simulink model "rc_coder"  (R2019b)
settings: Solver=FixedStepDiscrete  StartTime=0.0  StopTime=Inf  FixedStep=0.025  RelTol=1e-3  EnableMultiTasking=on
PreLoadFcn:
  | mdlname = bdroot;
  | oldFolder = cd(fileparts(which(mdlname)));
  | % cd ..\
  | 
  | load('./bus_type/bus_type.mat');
model workspace (MAT data in the model file):
  ADCDRES : Simulink.Parameter (value not decoded)
  ADCSRES : Simulink.Parameter (value not decoded)
  CLK : Simulink.Parameter (value not decoded)
  EncoderScaler : Simulink.Parameter (value not decoded)
  GearBoxScaler : Simulink.Parameter (value not decoded)
  Kd_T : Simulink.Parameter (value not decoded)
  Kd_theta : Simulink.Parameter (value not decoded)
  Ki_T : Simulink.Parameter (value not decoded)
  Ki_theta : Simulink.Parameter (value not decoded)
  Kp_T : Simulink.Parameter (value not decoded)
  Kp_theta : Simulink.Parameter (value not decoded)
  LowerTempLimitHigh : Simulink.Parameter (value not decoded)
  LowerTempLimitLow : Simulink.Parameter (value not decoded)
  MinMeasurableSpd : Simulink.Parameter (value not decoded)
  ModePWM : Simulink.Parameter (value not decoded)
  ModePosition : Simulink.Parameter (value not decoded)
  ModePrecool : Simulink.Parameter (value not decoded)
  ModeTemp : Simulink.Parameter (value not decoded)
  PWMFreq : Simulink.Parameter (value not decoded)
  QuadratureEncScaler : Simulink.Parameter (value not decoded)
  S1DelaySeconds : Simulink.Parameter (value not decoded)
  S2DelaySeconds : Simulink.Parameter (value not decoded)
  S3DelaySeconds : Simulink.Parameter (value not decoded)
  S4DelaySeconds : Simulink.Parameter (value not decoded)
  SamplingR : Simulink.Parameter (value not decoded)
  StepSize : Simulink.Parameter (value not decoded)
  TErrBand : Simulink.Parameter (value not decoded)
  ThetaErrBand : Simulink.Parameter (value not decoded)
  VADCREF : Simulink.Parameter (value not decoded)
symbols that are objects in the model workspace (value not decoded): ADCDRES, CLK, EncoderScaler, GearBoxScaler, Kd_T, Kd_theta, Ki_T, Ki_theta, Kp_T, Kp_theta, LowerTempLimitHigh, LowerTempLimitLow, MinMeasurableSpd, ModePosition, ModePrecool, ModePWM, ModeTemp, PWMFreq, QuadratureEncScaler, S1DelaySeconds, S2DelaySeconds, S3DelaySeconds, S4DelaySeconds, StepSize, TErrBand, ThetaErrBand
undefined symbols (not defined in the file or in its folder): DiscIntNeverNeededParam, Down, GPTRIP1SEL, GPTRIP2SEL, TZ1, TZ2, Up
libraries: simulink x21, c2802xlib x12, c2837xDlib x10, c280xlib x9, dspstat3 x8, dspfdesign x7, commutil2 x3, c2000lib x2
(part 2 of 4)

== system rc_coder/Controller/Precool Mode ==
  Cmd : Inport
  Action Port : ActionPort  ActionPortLabel=case [ 60 ]:
  Bit to Integer Converter : commutil2/Bit to Integer Converter  nbits=4  bitOrder=MSB first  signedOutputValues=Unsigned  outDtype=Inherit via internal rule  outDtypeSigned=Inherit via internal rule
      settings: SourceProductName=Communications Toolbox
  Bus Selector : BusSelector  OutputSignals=Cmd1,Cmd2,Cmd3,Cmd4
  Constant : Constant  Value=0  OutDataTypeStr=single
  Mux : Mux
  s1 : Outport
  s2 : Outport  Port=2
  s3 : Outport  Port=3
  s4 : Outport  Port=4
  valve : Outport  Port=5
  wires:
  Constant/1 -> s4/1, s3/1, s2/1, s1/1
  Cmd/1 -> Bus Selector/1
  Bit to Integer Converter/1 -> valve/1
  Mux/1 -> Bit to Integer Converter/1
  Bus Selector/1 -> Mux/1  "<Cmd1>"
  Bus Selector/2 -> Mux/2  "<Cmd2>"
  Bus Selector/3 -> Mux/3  "<Cmd3>"
  Bus Selector/4 -> Mux/4  "<Cmd4>"

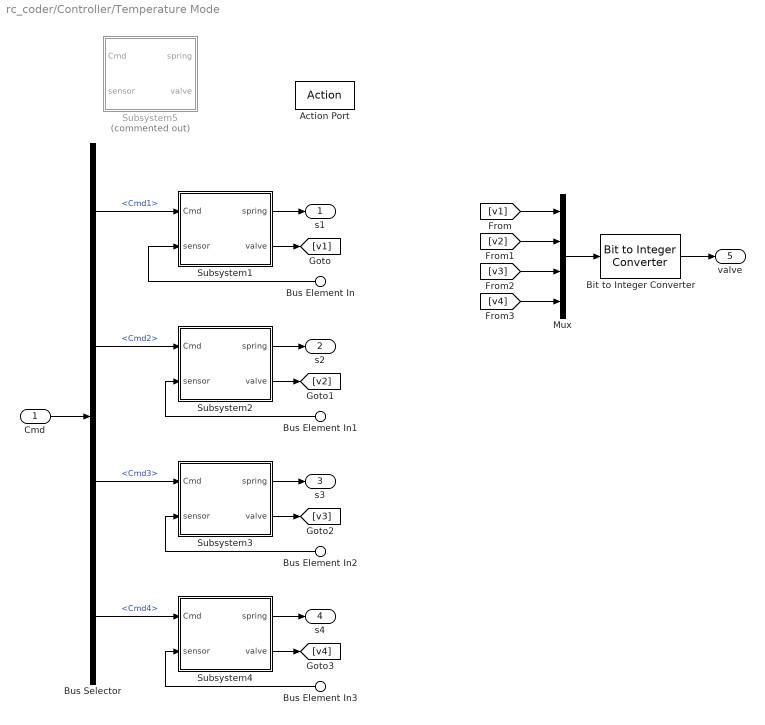
== system rc_coder/Controller/Temperature Mode ==
  Cmd : Inport
  Bus Element In : Inport  Port=2  PortName=feedback  Element=T.T1
  Bus Element In1 : Inport  Port=2  PortName=feedback  Element=T.T2
  Bus Element In2 : Inport  Port=2  PortName=feedback  Element=T.T3
  Bus Element In3 : Inport  Port=2  PortName=feedback  Element=T.T4
  Action Port : ActionPort  ActionPortLabel=case [ 55 ]:
  Bit to Integer Converter : commutil2/Bit to Integer Converter  nbits=4  bitOrder=MSB first  signedOutputValues=Unsigned  outDtype=Inherit via internal rule  outDtypeSigned=Inherit via internal rule
      settings: SourceProductName=Communications Toolbox
  Bus Selector : BusSelector  OutputSignals=Cmd1,Cmd2,Cmd3,Cmd4
  Mux : Mux
  Subsystem1 : Subsystem
  Subsystem2 : Subsystem
  Subsystem3 : Subsystem
  Subsystem4 : Subsystem
  Subsystem5 : Subsystem  Commented=on
  s1 : Outport
  s2 : Outport  Port=2
  s3 : Outport  Port=3
  s4 : Outport  Port=4
  valve : Outport  Port=5
  wires:
  Cmd/1 -> Bus Selector/1
  Subsystem2/1(spring) -> s2/1
  Subsystem3/1(spring) -> s3/1
  Bus Element In3/1 -> Subsystem4/2(sensor)
  Bus Selector/4 -> Subsystem4/1(Cmd)  "<Cmd4>"
  Subsystem4/1(spring) -> s4/1
  Bus Element In2/1 -> Subsystem3/2(sensor)
  Bus Selector/3 -> Subsystem3/1(Cmd)  "<Cmd3>"
  Mux/1 -> Bit to Integer Converter/1
  [v1] -> Mux/1
  [v2] -> Mux/2
  [v3] -> Mux/3
  [v4] -> Mux/4
  Bit to Integer Converter/1 -> valve/1
  Bus Selector/1 -> Subsystem1/1(Cmd)  "<Cmd1>"
  Bus Element In/1 -> Subsystem1/2(sensor)
  Subsystem1/1(spring) -> s1/1
  Subsystem1/2(valve) -> [v1]
  Bus Selector/2 -> Subsystem2/1(Cmd)  "<Cmd2>"
  Subsystem2/2(valve) -> [v2]
  Bus Element In1/1 -> Subsystem2/2(sensor)
  Subsystem3/2(valve) -> [v3]
  Subsystem4/2(valve) -> [v4]

== system rc_coder/Data Uploading/Subsystem1 ==
  In1 : Inport
  Constant2 : Constant  Value=f
  Data Type Conversion : DataTypeConversion  OutDataTypeStr=int32
  Product1 : Product
  Rounding Function : Rounding  Operator=round
  Out1 : Outport
  wires:
  Rounding Function/1 -> Data Type Conversion/1
  Constant2/1 -> Product1/2
  In1/1 -> Product1/1
  Product1/1 -> Rounding Function/1
  Data Type Conversion/1 -> Out1/1

== system rc_coder/Data Uploading/Subsystem2 ==
  In1 : Inport
  Constant2 : Constant  Value=f
  Data Type Conversion : DataTypeConversion  OutDataTypeStr=int32
  Product1 : Product
  Rounding Function : Rounding  Operator=round
  Out1 : Outport
  wires:
  Data Type Conversion/1 -> Out1/1
  Product1/1 -> Rounding Function/1
  In1/1 -> Product1/1
  Constant2/1 -> Product1/2
  Rounding Function/1 -> Data Type Conversion/1

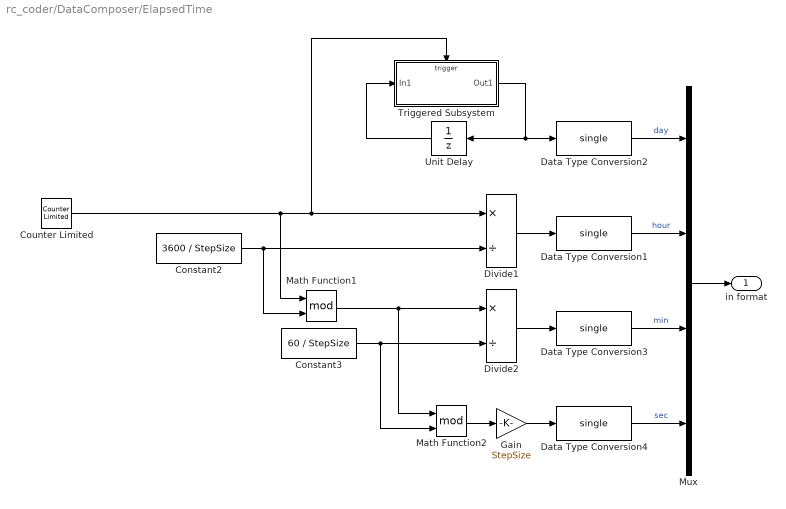
== system rc_coder/DataComposer/ElapsedTime ==
  Constant2 : Constant  Value=3600 / StepSize  OutDataTypeStr=uint32
  Constant3 : Constant  Value=60 / StepSize  OutDataTypeStr=uint32
  Counter Limited : simulink/Sources/Counter Limited  uplimit=1 / StepSize * 60 * 60 * 24  tsamp=-1
  Data Type Conversion{1..4} (4 alike) : DataTypeConversion  OutDataTypeStr=single
  Divide1 : Product  Inputs=*/  OutDataTypeStr=uint8
  Divide2 : Product  Inputs=*/  OutDataTypeStr=uint8
  Gain : Gain  Gain=StepSize  OutDataTypeStr=single
  Math Function1 : Math  Operator=mod  SignedPower=off  SaturateOnIntegerOverflow=on
  Math Function2 : Math  Operator=mod  SignedPower=off  SaturateOnIntegerOverflow=on
  Mux : Mux
  Triggered Subsystem : Subsystem  TreatAsAtomicUnit=on
  Unit Delay : UnitDelay  SampleTime=-1  HasFrameUpgradeWarning=on
  in format : Outport
  wires:
  Counter Limited/1 -> Divide1/1, Triggered Subsystem/Trigger, Math Function1/1
  Divide1/1 -> Data Type Conversion1/1
  Divide2/1 -> Data Type Conversion3/1
  Constant2/1 -> Math Function1/2, Divide1/2
  Math Function1/1 -> Divide2/1, Math Function2/1
  Data Type Conversion2/1 -> Mux/1  "day"
  Data Type Conversion1/1 -> Mux/2  "hour"
  Data Type Conversion3/1 -> Mux/3  "min"
  Data Type Conversion4/1 -> Mux/4  "sec"
  Math Function2/1 -> Gain/1
  Constant3/1 -> Divide2/2, Math Function2/2
  Mux/1 -> in format/1
  Triggered Subsystem/1(Out1) -> Data Type Conversion2/1, Unit Delay/1
  Unit Delay/1 -> Triggered Subsystem/1(In1)
  Gain/1 -> Data Type Conversion4/1

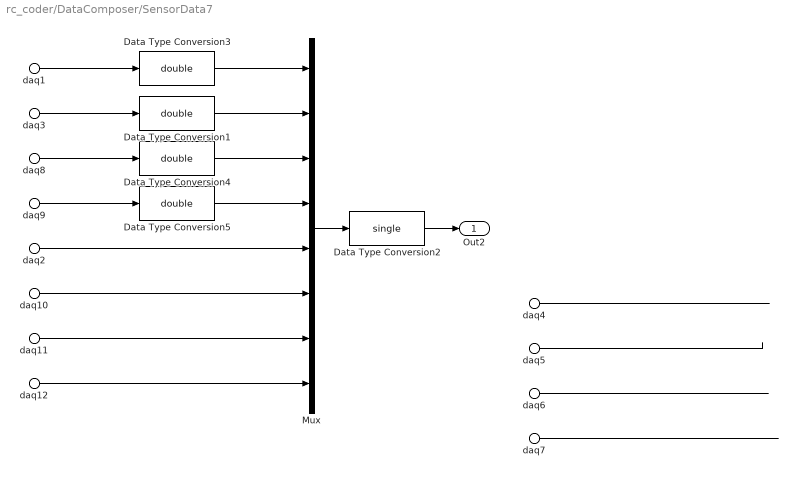
== system rc_coder/DataComposer/SensorData7 ==
  daq1 : Inport  PortName=daq  Element=ENC.PosA
  daq3 : Inport  PortName=daq  Element=ENC.SpdA
  daq8 : Inport  PortName=daq  Element=ENC.PosB
  daq9 : Inport  PortName=daq  Element=ENC.SpdB
  daq2 : Inport  PortName=daq  Element=T.T1
  daq10 : Inport  PortName=daq  Element=T.T2
  daq11 : Inport  PortName=daq  Element=T.T3
  daq12 : Inport  PortName=daq  Element=T.T4
  daq4 : Inport  PortName=daq  Element=I.current1
  daq5 : Inport  PortName=daq  Element=I.current2
  daq6 : Inport  PortName=daq  Element=I.current3
  daq7 : Inport  PortName=daq  Element=I.current4
  Data Type Conversion{1,3..5} (4 alike) : DataTypeConversion  OutDataTypeStr=double
  Data Type Conversion2 : DataTypeConversion  OutDataTypeStr=single
  Mux : Mux  Inputs=8
  Out2 : Outport
  wires:
  daq3/1 -> Data Type Conversion1/1
  Data Type Conversion1/1 -> Mux/2
  Data Type Conversion3/1 -> Mux/1
  daq2/1 -> Mux/5
  daq1/1 -> Data Type Conversion3/1
  Mux/1 -> Data Type Conversion2/1
  daq4/1 -> ?
  daq5/1 -> ?
  daq6/1 -> ?
  daq7/1 -> ?
  Data Type Conversion2/1 -> Out2/1
  daq8/1 -> Data Type Conversion4/1
  Data Type Conversion4/1 -> Mux/3
  daq9/1 -> Data Type Conversion5/1
  Data Type Conversion5/1 -> Mux/4
  daq10/1 -> Mux/6
  daq11/1 -> Mux/7
  daq12/1 -> Mux/8

== system rc_coder/Receive/Triggered Subsystem2 ==
  SCIA RCV Interrupt : TriggerPort  TriggerType=function-call  VariantControl=Variant
  SCI Receive : c280xlib/SCI Receive  sciModule=B  dataHead=''  dataTail=''  dataType=single  dataDim=5  initValue=0  errOption=Output the last received value  errValue=0  sampleTime=-1  outputStatus=off  postInterrupt=on  numFifo=1
      settings: SourceProductName=Embedded Coder Support Package for Texas Instruments C2000 Processors  SourceProductBaseCode=TIC2000
  Serial Command : Outport
  wires:
  SCI Receive/1 -> Serial Command/1

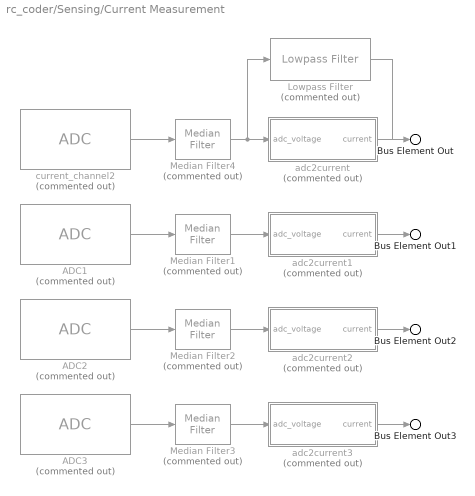
== system rc_coder/Sensing/Current Measurement ==
  ADC1 : c2802xlib/ADC  Commented=on  blkParamProc=C2000_Type4  ADCModule=B  samplingMode=Single sample mode  ADCResolution=16-bit (Differential inputs)  useSOC1=SOC5  useSOC2=SOC0_SOC1  SOCAcquisitionWindow=15  SOCTriggerSource=Software  SOCInterruptTrigger=No ADCINT  Ts=-1  dType=double  postInterrupt=off  interruptSel=ADCINT1  ADCINTContinuous=on  endma=off  chdma=1  conv1=ADCINA0  conv2=ADCINA0 and ADCINB0  conv1_Type4=ADCIN5  conv2_Type4=ADCIN4 and ADCIN5
      settings: SourceProductName=Embedded Coder Support Package for Texas Instruments C2000 Processors
  ADC2 : c2802xlib/ADC  Commented=on  blkParamProc=C2000_Type4  ADCModule=C  samplingMode=Single sample mode  ADCResolution=16-bit (Differential inputs)  useSOC1=SOC5  useSOC2=SOC0_SOC1  SOCAcquisitionWindow=15  SOCTriggerSource=Software  SOCInterruptTrigger=No ADCINT  Ts=-1  dType=double  postInterrupt=off  interruptSel=ADCINT1  ADCINTContinuous=on  endma=off  chdma=1  conv1=ADCINA0  conv2=ADCINA0 and ADCINB0  conv1_Type4=ADCIN5  conv2_Type4=ADCIN4 and ADCIN5
      settings: SourceProductName=Embedded Coder Support Package for Texas Instruments C2000 Processors
  ADC3 : c2802xlib/ADC  Commented=on  blkParamProc=C2000_Type4  ADCModule=A  samplingMode=Single sample mode  ADCResolution=16-bit (Differential inputs)  useSOC1=SOC4  useSOC2=SOC0_SOC1  SOCAcquisitionWindow=15  SOCTriggerSource=Software  SOCInterruptTrigger=No ADCINT  Ts=-1  dType=double  postInterrupt=off  interruptSel=ADCINT1  ADCINTContinuous=on  endma=off  chdma=1  conv1=ADCINA0  conv2=ADCINA0 and ADCINB0  conv1_Type4=ADCIN4  conv2_Type4=ADCIN0 and ADCIN1
      settings: SourceProductName=Embedded Coder Support Package for Texas Instruments C2000 Processors
  Lowpass Filter : dspfdesign/Lowpass Filter  Commented=on  FilterType=FIR  DesignForMinimumOrder=on  FilterOrder=50  PassbandFrequency=2  StopbandFrequency=5  PassbandRipple=0.1  StopbandAttenuation=80  InheritSampleRate=off  SampleRate=1000  SimulateUsing=Code generation  roundingMode=Floor  coeffsDataTypeStr=fixdt(1,16)
  Median Filter1 : dspstat3/Median Filter  Commented=on  WindowLength=5  SimulateUsing=Code generation
      settings: SourceProductName=DSP System Toolbox  SourceProductBaseCode=DS
  Median Filter2 : dspstat3/Median Filter  Commented=on  WindowLength=5  SimulateUsing=Code generation
      settings: SourceProductName=DSP System Toolbox  SourceProductBaseCode=DS
  Median Filter3 : dspstat3/Median Filter  Commented=on  WindowLength=5  SimulateUsing=Code generation
      settings: SourceProductName=DSP System Toolbox  SourceProductBaseCode=DS
  Median Filter4 : dspstat3/Median Filter  Commented=on  WindowLength=10  SimulateUsing=Code generation
      settings: SourceProductName=DSP System Toolbox  SourceProductBaseCode=DS
  adc2current : Subsystem  Commented=on
  adc2current1 : Subsystem  Commented=on
  adc2current2 : Subsystem  Commented=on
  adc2current3 : Subsystem  Commented=on
  current_channel2 : c2802xlib/ADC  Commented=on  blkParamProc=C2000_Type4  ADCModule=A  samplingMode=Single sample mode  ADCResolution=16-bit (Differential inputs)  useSOC1=SOC2  useSOC2=SOC0_SOC1  SOCAcquisitionWindow=15  SOCTriggerSource=Software  SOCInterruptTrigger=No ADCINT  Ts=-1  dType=double  postInterrupt=off  interruptSel=ADCINT1  ADCINTContinuous=on  endma=off  chdma=1  conv1=ADCINA0  conv2=ADCINA0 and ADCINB0  conv1_Type4=ADCIN5  conv2_Type4=ADCIN4 and ADCIN5
      settings: SourceProductName=Embedded Coder Support Package for Texas Instruments C2000 Processors
  Bus Element Out : Outport  PortName=OutBus  Element=current1
  Bus Element Out1 : Outport  PortName=OutBus  Element=current2
  Bus Element Out2 : Outport  PortName=OutBus  Element=current3
  Bus Element Out3 : Outport  PortName=OutBus  Element=current4
  wires:
  ADC1/1 -> Median Filter1/1
  current_channel2/1 -> Median Filter4/1
  ADC2/1 -> Median Filter2/1
  ADC3/1 -> Median Filter3/1
  adc2current1/1(current) -> Bus Element Out1/1
  adc2current2/1(current) -> Bus Element Out2/1
  adc2current3/1(current) -> Bus Element Out3/1
  Median Filter1/1 -> adc2current1/1(adc_voltage)
  Median Filter2/1 -> adc2current2/1(adc_voltage)
  Median Filter3/1 -> adc2current3/1(adc_voltage)
  Median Filter4/1 -> Lowpass Filter/1, adc2current/1(adc_voltage)
  adc2current/1(current) -> ?
  Lowpass Filter/1 -> Bus Element Out/1

== system rc_coder/Sensing/Incremental Encoder ==
  CalcSpd : Subsystem
  CalcSpd1 : Subsystem
  Gain1 : Gain  Gain=360 / (EncoderScaler * GearBoxScaler * QuadratureEncScaler)
  Gain2 : Gain  Gain=360 / (EncoderScaler * GearBoxScaler * QuadratureEncScaler)
  eCAP : c280xlib/eCAP  operatingMode=eCAP  selectCAPx=eCAP1  offsetValue=0  counterSynIn=off  enableCounter=off  syncOutput=Disabled  sampleTime=-1  eventPrescaler=0  selectMode=Continuous  enableOneShot=off  stopValue=Capture Event 1  resetEv1Ts=on  ev1Polarity=Rising Edge  resetEv2Ts=off  ev2Polarity=Rising Edge  resetEv3Ts=off  ev3Polarity=Rising Edge  resetEv4Ts=off  ev4Polarity=Rising Edge  tSCntrDataType=uint32  capEvFlag=off  capFlagDataType=uint16  overFlowFlag=on  overFlowFlagDataType=uint32  periodUnit=Seconds  periodSource=Specify via dialog  waveformPeriod=0.001  dutyUnit=Percentages  dutySource=Specify via dialog  dutyCycle=50  outputPolarity=Active High  enableCEVT1Int=off  enableCEVT2Int=off  enableCEVT3Int=off  enableCEVT4Int=off  enableCTROVFInt=off  enablePRDInt=off  enableCMPInt=off
      settings: SourceProductName=Embedded Coder Support Package for Texas Instruments C2000 Processors  SourceProductBaseCode=TIC2000
  eCAP1 : c280xlib/eCAP  operatingMode=eCAP  selectCAPx=eCAP4  offsetValue=0  counterSynIn=off  enableCounter=off  syncOutput=Disabled  sampleTime=-1  eventPrescaler=0  selectMode=Continuous  enableOneShot=off  stopValue=Capture Event 1  resetEv1Ts=on  ev1Polarity=Rising Edge  resetEv2Ts=off  ev2Polarity=Rising Edge  resetEv3Ts=off  ev3Polarity=Rising Edge  resetEv4Ts=off  ev4Polarity=Rising Edge  tSCntrDataType=uint32  capEvFlag=off  capFlagDataType=uint16  overFlowFlag=on  overFlowFlagDataType=uint32  periodUnit=Seconds  periodSource=Specify via dialog  waveformPeriod=0.001  dutyUnit=Percentages  dutySource=Specify via dialog  dutyCycle=50  outputPolarity=Active High  enableCEVT1Int=off  enableCEVT2Int=off  enableCEVT3Int=off  enableCEVT4Int=off  enableCTROVFInt=off  enablePRDInt=off  enableCMPInt=off
      settings: SourceProductName=Embedded Coder Support Package for Texas Instruments C2000 Processors  SourceProductBaseCode=TIC2000
  eQEP : c280xlib/eQEP  useModule=eQEP1  pcInputmode=Quadrature-count  externalClockrate=2x resolution: Count the rising/falling edge  swapPolarityselection=Clockwise  qdfOutputport=on  qapPolarityselection=off  qbpPolarityselection=off  qipPolarityselection=off  qspPolarityselection=off  igatePolarityselection=off  sampleTime=-1  pcOutputport=on  pcMaximumvalue=4294967295  indexInitializationcheck=off  indexInitializationevent=Rising edge  strobeInitializationcheck=off  strobeInitializationevent=Rising edge  softwareInitializationcheck=off  softwareInitializationsource=Set to init value at start up  softwareInitializationmode=on  pcInitialvalue=2147483648  pcResetmode=Reset on an index event  ieloutputport=off  indexEventlatch=Rising edge  seloutputport=off  strobeEventlatch=Rising edge  pcefOutputport=off  enableEqepcapture=off  qctmrOutputport=off  qcprdOutputport=off  captureTimerprescaler=128  upEventprescaler=2  overflowErrorflag=off  directionErrorflag=off  captureTimerposition=On position counter read  unitTimerperiod=100000000  captureTimerlatch=off  capturePeriodlatch=on  positionCounterlatch=off  soenPolarityselection=off  spselPolarityselection=Index pin is used for sync output  compareValuesource=Specify via dialog  shadowMode=Load on QPOSCNT=0  compareValue=4294967295  syncOutputwidth=1  polaritySyncoutput=Active high  watchdogEnable=off  watchdogTimer=65535  outport1Datatype=auto  outport2Datatype=int32  outport3Datatype=auto  outport4Datatype=auto  outport5Datatype=auto  outport6Datatype=auto  outport7Datatype=auto  outport8Datatype=auto  outport9Datatype=auto  outport10Datatype=auto  outport11Datatype=auto  outport12Datatype=auto  eqepinterrupt_pce=off  eqepinterrupt_qpe=off  eqepinterrupt_qdc=off  eqepinterrupt_wto=off  eqepinterrupt_pcu=off  eqepinterrupt_pco=off  eqepinterrupt_pcr=off  eqepinterrupt_pcm=off  eqepinterrupt_sel=off  eqepinterrupt_iel=off  eqepinterrupt_uto=off  pheOutputport=off  watchdogOutputport=off  outport13Datatype=auto  outport14Datatype=auto
      settings: SourceProductName=Embedded Coder Support Package for Texas Instruments C2000 Processors  SourceProductBaseCode=TIC2000
  eQEP1 : c280xlib/eQEP  useModule=eQEP2  pcInputmode=Quadrature-count  externalClockrate=2x resolution: Count the rising/falling edge  swapPolarityselection=Clockwise  qdfOutputport=on  qapPolarityselection=off  qbpPolarityselection=off  qipPolarityselection=off  qspPolarityselection=off  igatePolarityselection=off  sampleTime=-1  pcOutputport=on  pcMaximumvalue=4294967295  indexInitializationcheck=off  indexInitializationevent=Rising edge  strobeInitializationcheck=off  strobeInitializationevent=Rising edge  softwareInitializationcheck=off  softwareInitializationsource=Set to init value at start up  softwareInitializationmode=on  pcInitialvalue=2147483648  pcResetmode=Reset on an index event  ieloutputport=off  indexEventlatch=Rising edge  seloutputport=off  strobeEventlatch=Rising edge  pcefOutputport=off  enableEqepcapture=off  qctmrOutputport=off  qcprdOutputport=on  captureTimerprescaler=128  upEventprescaler=128  overflowErrorflag=off  directionErrorflag=off  captureTimerposition=On position counter read  unitTimerperiod=100000000  captureTimerlatch=off  capturePeriodlatch=off  positionCounterlatch=off  soenPolarityselection=off  spselPolarityselection=Index pin is used for sync output  compareValuesource=Specify via dialog  shadowMode=Load on QPOSCNT=0  compareValue=4294967295  syncOutputwidth=1  polaritySyncoutput=Active high  watchdogEnable=off  watchdogTimer=65535  outport1Datatype=auto  outport2Datatype=int32  outport3Datatype=auto  outport4Datatype=auto  outport5Datatype=auto  outport6Datatype=auto  outport7Datatype=auto  outport8Datatype=auto  outport9Datatype=auto  outport10Datatype=auto  outport11Datatype=auto  outport12Datatype=auto  eqepinterrupt_pce=off  eqepinterrupt_qpe=off  eqepinterrupt_qdc=off  eqepinterrupt_wto=off  eqepinterrupt_pcu=off  eqepinterrupt_pco=off  eqepinterrupt_pcr=off  eqepinterrupt_pcm=off  eqepinterrupt_sel=off  eqepinterrupt_iel=off  eqepinterrupt_uto=off  pheOutputport=off  watchdogOutputport=off  outport13Datatype=auto  outport14Datatype=auto
      settings: SourceProductName=Embedded Coder Support Package for Texas Instruments C2000 Processors  SourceProductBaseCode=TIC2000
  Bus Element Out : Outport  PortName=OutBus  Element=PosA
  Bus Element Out1 : Outport  PortName=OutBus  Element=SpdA
  Bus Element Out2 : Outport  PortName=OutBus  Element=PosB
  Bus Element Out3 : Outport  PortName=OutBus  Element=SpdB
  wires:
  eQEP/2 -> Gain1/1, CalcSpd/2(qposcnt)
  Gain1/1 -> Bus Element Out/1
  eQEP1/1 -> CalcSpd1/1(dir)
  eQEP1/2 -> Gain2/1, CalcSpd1/2(qposcnt)
  Gain2/1 -> Bus Element Out2/1
  CalcSpd/1(speed) -> Bus Element Out1/1
  eCAP/1 -> CalcSpd/3(qcprd)
  eCAP/2 -> CalcSpd/4(overflow)
  eQEP/1 -> CalcSpd/1(dir)
  CalcSpd1/1(speed) -> Bus Element Out3/1
  eCAP1/1 -> CalcSpd1/3(qcprd)
  eCAP1/2 -> CalcSpd1/4(overflow)

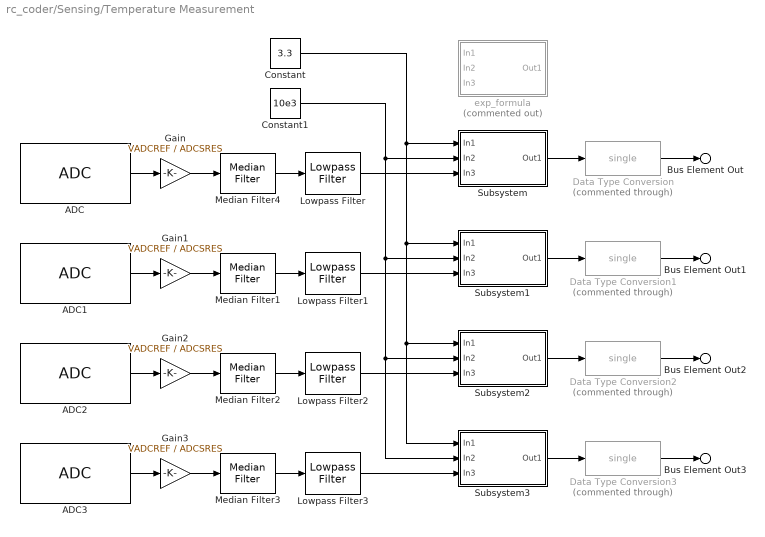
== system rc_coder/Sensing/Temperature Measurement ==
  ADC : c2802xlib/ADC  blkParamProc=C2000_Type4  ADCModule=C  samplingMode=Single sample mode  ADCResolution=12-bit (Single-ended input)  useSOC1=SOC3  useSOC2=SOC0_SOC1  SOCAcquisitionWindow=15  SOCTriggerSource=Software  SOCInterruptTrigger=No ADCINT  Ts=-1  dType=double  postInterrupt=off  interruptSel=ADCINT1  ADCINTContinuous=on  endma=off  chdma=1  conv1=ADCINA0  conv2=ADCINA0 and ADCINB0  conv1_Type4=ADCIN3  conv2_Type4=ADCIN2 and ADCIN3
      settings: SourceProductName=Embedded Coder Support Package for Texas Instruments C2000 Processors
  ADC1 : c2802xlib/ADC  blkParamProc=C2000_Type4  ADCModule=B  samplingMode=Single sample mode  ADCResolution=12-bit (Single-ended input)  useSOC1=SOC3  useSOC2=SOC0_SOC1  SOCAcquisitionWindow=15  SOCTriggerSource=Software  SOCInterruptTrigger=No ADCINT  Ts=-1  dType=double  postInterrupt=off  interruptSel=ADCINT1  ADCINTContinuous=on  endma=off  chdma=1  conv1=ADCINA0  conv2=ADCINA0 and ADCINB0  conv1_Type4=ADCIN3  conv2_Type4=ADCIN0 and ADCIN1
      settings: SourceProductName=Embedded Coder Support Package for Texas Instruments C2000 Processors
  ADC2 : c2802xlib/ADC  blkParamProc=C2000_Type4  ADCModule=A  samplingMode=Single sample mode  ADCResolution=12-bit (Single-ended input)  useSOC1=SOC3  useSOC2=SOC0_SOC1  SOCAcquisitionWindow=15  SOCTriggerSource=Software  SOCInterruptTrigger=No ADCINT  Ts=-1  dType=double  postInterrupt=off  interruptSel=ADCINT1  ADCINTContinuous=on  endma=off  chdma=1  conv1=ADCINA0  conv2=ADCINA0 and ADCINB0  conv1_Type4=ADCIN3  conv2_Type4=ADCIN0 and ADCIN1
      settings: SourceProductName=Embedded Coder Support Package for Texas Instruments C2000 Processors
  ADC3 : c2802xlib/ADC  blkParamProc=C2000_Type4  ADCModule=C  samplingMode=Single sample mode  ADCResolution=12-bit (Single-ended input)  useSOC1=SOC2  useSOC2=SOC0_SOC1  SOCAcquisitionWindow=15  SOCTriggerSource=Software  SOCInterruptTrigger=No ADCINT  Ts=-1  dType=double  postInterrupt=off  interruptSel=ADCINT1  ADCINTContinuous=on  endma=off  chdma=1  conv1=ADCINA0  conv2=ADCINA0 and ADCINB0  conv1_Type4=ADCIN2  conv2_Type4=ADCIN0 and ADCIN1
      settings: SourceProductName=Embedded Coder Support Package for Texas Instruments C2000 Processors
  Constant : Constant  Value=3.3  OutDataTypeStr=double
  Constant1 : Constant  Value=10e3  OutDataTypeStr=double
  Data Type Conversion{,1..3} (4 alike) : DataTypeConversion  Commented=through  OutDataTypeStr=single
  Gain{,1..3} (4 alike) : Gain  Gain=VADCREF / ADCSRES
  Lowpass Filter{,1..3} (4 alike) : dspfdesign/Lowpass Filter  FilterType=IIR  DesignForMinimumOrder=on  FilterOrder=50  PassbandFrequency=10  StopbandFrequency=19  PassbandRipple=0.1  StopbandAttenuation=80  InheritSampleRate=off  SampleRate=1/StepSize  SimulateUsing=Code generation  roundingMode=Floor  coeffsDataTypeStr=fixdt(1,16)
  Median Filter{1..4} (4 alike) : dspstat3/Median Filter  WindowLength=5  SimulateUsing=Code generation
      settings: SourceProductName=DSP System Toolbox  SourceProductBaseCode=DS
  Subsystem : Subsystem
      mask Display:
      | disp('u2T');
      | port_label('input', 1, 'excitation');
      | port_label('input', 2, 'R');
      | port_label('input', 3, 'u');
  Subsystem1 : Subsystem
      mask Display:
      | disp('u2T');
      | port_label('input', 1, 'excitation');
      | port_label('input', 2, 'R');
      | port_label('input', 3, 'u');
  Subsystem2 : Subsystem
      mask Display:
      | disp('u2T');
      | port_label('input', 1, 'excitation');
      | port_label('input', 2, 'R');
      | port_label('input', 3, 'u');
  Subsystem3 : Subsystem
      mask Display:
      | disp('u2T');
      | port_label('input', 1, 'excitation');
      | port_label('input', 2, 'R');
      | port_label('input', 3, 'u');
  exp_formula : Subsystem  Commented=on
      mask Display:
      | disp('u2T');
      | port_label('input', 1, 'excitation');
      | port_label('input', 2, 'R');
      | port_label('input', 3, 'u');
  Bus Element Out : Outport  PortName=OutBus  Element=T1
  Bus Element Out1 : Outport  PortName=OutBus  Element=T2
  Bus Element Out2 : Outport  PortName=OutBus  Element=T3
  Bus Element Out3 : Outport  PortName=OutBus  Element=T4
  wires:
  Subsystem1/1(Out1) -> Data Type Conversion1/1
  Gain1/1 -> Median Filter1/1
  Subsystem2/1(Out1) -> Data Type Conversion2/1
  Gain2/1 -> Median Filter2/1
  Median Filter1/1 -> Lowpass Filter1/1
  Median Filter2/1 -> Lowpass Filter2/1
  ADC/1 -> Gain/1
  Median Filter4/1 -> Lowpass Filter/1
  Median Filter3/1 -> Lowpass Filter3/1
  Constant1/1 -> Subsystem1/2(In2), Subsystem3/2(In2), Subsystem2/2(In2), Subsystem/2(In2)
  Gain3/1 -> Median Filter3/1
  Subsystem3/1(Out1) -> Data Type Conversion3/1
  Lowpass Filter/1 -> Subsystem/3(In3)
  Lowpass Filter1/1 -> Subsystem1/3(In3)
  Lowpass Filter2/1 -> Subsystem2/3(In3)
  Lowpass Filter3/1 -> Subsystem3/3(In3)
  Gain/1 -> Median Filter4/1
  ADC3/1 -> Gain3/1
  ADC2/1 -> Gain2/1
  ADC1/1 -> Gain1/1
  Data Type Conversion/1 -> Bus Element Out/1
  Data Type Conversion1/1 -> Bus Element Out1/1
  Data Type Conversion2/1 -> Bus Element Out2/1
  Data Type Conversion3/1 -> Bus Element Out3/1
  Subsystem/1(Out1) -> Data Type Conversion/1
  Constant/1 -> Subsystem/1(In1), Subsystem1/1(In1), Subsystem3/1(In1), Subsystem2/1(In1)

== system rc_coder/SerialCommInterface1/Triggered Subsystem1 ==
  TX : Inport
  SCIA RCV Interrupt : TriggerPort  TriggerType=function-call  VariantControl=Variant
  Mux : Mux  Inputs=2
  SCI Receive : c280xlib/SCI Receive  sciModule=A  dataHead=''  dataTail=''  dataType=single  dataDim=1  initValue=0  errOption=Output the last received value  errValue=0  sampleTime=-1  outputStatus=off  postInterrupt=on  numFifo=1
      settings: SourceProductName=Embedded Coder Support Package for Texas Instruments C2000 Processors  SourceProductBaseCode=TIC2000
  SCI Transmit : c280xlib/SCI Transmit  sciModule=A  dataHead=''  dataTail=''  postInterrupt=off  numFifo=1
      settings: SourceProductName=Embedded Coder Support Package for Texas Instruments C2000 Processors
  Serial Command : Outport
  wires:
  TX/1 -> Mux/2
  Mux/1 -> SCI Transmit/1
  SCI Receive/1 -> Mux/1, Serial Command/1

== system rc_coder/Transmit/DataFlowSwitch ==
  status : Inport
  If Action Subsystem1 : Subsystem  TreatAsAtomicUnit=on
  If Action Subsystem2 : Subsystem  TreatAsAtomicUnit=on
  If1 : If  IfExpression=(u1 == ModePosition) | (u1 == ModePrecool) | (u1 == ModePWM) | (u1 == ModeTemp)
  If2 : If  Commented=on  IfExpression=(u1 == ModePosition) | (u1 == ModePrecool)
  Merge : Merge
  switch : Outport
  wires:
  If Action Subsystem1/1(Out1) -> Merge/1
  If Action Subsystem2/1(Out1) -> Merge/2
  If1/2 -> If Action Subsystem2/Action
  Merge/1 -> switch/1
  If1/1 -> If Action Subsystem1/Action
  status/1 -> If1/1, If Action Subsystem2/1(In1)

== system rc_coder/Transmit/If Action Subsystem ==
  received : Inport
  status : Inport  Port=2
  data : Inport  Port=3
  Action Port : ActionPort  ActionPortLabel=if(u1 == 1)
  Mux : Mux  Inputs=3
  SCI Transmit : c280xlib/SCI Transmit  sciModule=B  dataHead=''  dataTail=''  postInterrupt=off  numFifo=1
      settings: SourceProductName=Embedded Coder Support Package for Texas Instruments C2000 Processors
  wires:
  status/1 -> Mux/2
  data/1 -> Mux/3
  Mux/1 -> SCI Transmit/1
  received/1 -> Mux/1

== system rc_coder/Controller/Position Mode/PID ==
  note: integrator and derivative should be of discrete type due to descrete solver
  In1 : Inport
  In2 : Inport  Port=2
  In3 : Inport  Port=3
  In4 : Inport  Port=4
  Abs : Abs
  Add : Sum  Inputs=+++
  Constant1 : Constant
  Constant5 : Constant  Value=0
  Discrete Derivative : simulink/Discrete/Discrete Derivative  gainval=1.0  ICPrevScaledInput=0.0  OutMin=[]  OutMax=[]  OutDataType=fixdt(1, 16)  OutScaling=2^-10  DoSatur=off
  Discrete-Time Integrator : DiscreteIntegrator  SampleTime=-1  LimitOutput=on  UpperSaturationLimit=0.5  LowerSaturationLimit=-0.5  ICPrevOutput=DiscIntNeverNeededParam  ICPrevScaledInput=DiscIntNeverNeededParam
  Product{,1..3} (4 alike) : Product
  Switch2 : Switch  Criteria=u2 > Threshold  Threshold=ThetaErrBand
  Out1 : Outport
  wires:
  Add/1 -> Product3/2
  Discrete Derivative/1 -> Add/3
  Discrete-Time Integrator/1 -> Add/2
  Product/1 -> Discrete-Time Integrator/1
  Product1/1 -> Discrete Derivative/1
  Product2/1 -> Add/1
  In1/1 -> Abs/1, Product2/1, Product/1, Product1/1
  Abs/1 -> Switch2/2
  Constant5/1 -> Switch2/3
  Product3/1 -> Out1/1
  Constant1/1 -> Switch2/1
  Switch2/1 -> Product3/1
  In2/1 -> Product2/2
  In3/1 -> Product/2
  In4/1 -> Product1/2

== system rc_coder/Controller/Position Mode/PID1 ==
  note: integrator and derivative should be of discrete type due to descrete solver
  In1 : Inport
  In2 : Inport  Port=2
  In3 : Inport  Port=3
  In4 : Inport  Port=4
  Abs : Abs
  Add : Sum  Inputs=+++
  Constant1 : Constant
  Constant5 : Constant  Value=0
  Discrete Derivative : simulink/Discrete/Discrete Derivative  gainval=1.0  ICPrevScaledInput=0.0  OutMin=[]  OutMax=[]  OutDataType=fixdt(1, 16)  OutScaling=2^-10  DoSatur=off
  Discrete-Time Integrator : DiscreteIntegrator  SampleTime=-1  LimitOutput=on  UpperSaturationLimit=0.5  LowerSaturationLimit=-0.5  ICPrevOutput=DiscIntNeverNeededParam  ICPrevScaledInput=DiscIntNeverNeededParam
  Product{,1..3} (4 alike) : Product
  Switch2 : Switch  Criteria=u2 > Threshold  Threshold=ThetaErrBand
  Out1 : Outport
  wires:
  In4/1 -> Product1/2
  In3/1 -> Product/2
  In2/1 -> Product2/2
  Switch2/1 -> Product3/1
  Constant1/1 -> Switch2/1
  Product3/1 -> Out1/1
  Constant5/1 -> Switch2/3
  Abs/1 -> Switch2/2
  In1/1 -> Product1/1, Product/1, Product2/1, Abs/1
  Product2/1 -> Add/1
  Product1/1 -> Discrete Derivative/1
  Product/1 -> Discrete-Time Integrator/1
  Discrete-Time Integrator/1 -> Add/2
  Discrete Derivative/1 -> Add/3
  Add/1 -> Product3/2

== system rc_coder/Controller/Position Mode/Subsystem1 ==
  Cmd : Inport
  sensor : Inport  Port=2
  Constant : Constant  Value=Kp_T
  Constant1 : Constant  Value=Ki_T
  Constant2 : Constant  Value=Kd_T
  Data Type Conversion : DataTypeConversion
  PID : Subsystem
  Saturation : Saturate  UpperLimit=60  LowerLimit=-20
  Subsystem : Subsystem
  Sum : Sum  Inputs=|+-
  spring : Outport
  valve : Outport  Port=2
  wires:
  Constant1/1 -> PID/3(Ki)
  Constant2/1 -> PID/4(Kd)
  Constant/1 -> PID/2(Kp)
  Cmd/1 -> Saturation/1
  Subsystem/1(heating) -> spring/1
  Subsystem/2(cooling) -> valve/1
  Data Type Conversion/1 -> PID/1(e)
  Saturation/1 -> Sum/1
  sensor/1 -> Sum/2
  PID/1(u) -> Subsystem/1(u)
  Sum/1 -> Data Type Conversion/1

== system rc_coder/Controller/Position Mode/Subsystem2 ==
  Cmd : Inport
  sensor : Inport  Port=2
  Constant : Constant  Value=Kp_T
  Constant1 : Constant  Value=Ki_T
  Constant2 : Constant  Value=Kd_T
  Data Type Conversion : DataTypeConversion
  PID : Subsystem
  Saturation : Saturate  UpperLimit=60  LowerLimit=-20
  Subsystem : Subsystem
  Sum : Sum  Inputs=|+-
  spring : Outport
  valve : Outport  Port=2
  wires:
  Sum/1 -> Data Type Conversion/1
  PID/1(u) -> Subsystem/1(u)
  sensor/1 -> Sum/2
  Saturation/1 -> Sum/1
  Data Type Conversion/1 -> PID/1(e)
  Subsystem/2(cooling) -> valve/1
  Subsystem/1(heating) -> spring/1
  Cmd/1 -> Saturation/1
  Constant/1 -> PID/2(Kp)
  Constant2/1 -> PID/4(Kd)
  Constant1/1 -> PID/3(Ki)

== system rc_coder/Controller/Position Mode/Subsystem3 ==
  Cmd : Inport
  sensor : Inport  Port=2
  Constant : Constant  Value=Kp_T
  Constant1 : Constant  Value=Ki_T
  Constant2 : Constant  Value=Kd_T
  Data Type Conversion : DataTypeConversion
  PID : Subsystem
  Saturation : Saturate  UpperLimit=60  LowerLimit=-20
  Subsystem : Subsystem
  Sum : Sum  Inputs=|+-
  spring : Outport
  valve : Outport  Port=2
  wires:
  Sum/1 -> Data Type Conversion/1
  PID/1(u) -> Subsystem/1(u)
  sensor/1 -> Sum/2
  Saturation/1 -> Sum/1
  Data Type Conversion/1 -> PID/1(e)
  Subsystem/2(cooling) -> valve/1
  Subsystem/1(heating) -> spring/1
  Cmd/1 -> Saturation/1
  Constant/1 -> PID/2(Kp)
  Constant2/1 -> PID/4(Kd)
  Constant1/1 -> PID/3(Ki)

== system rc_coder/Controller/Position Mode/Subsystem4 ==
  Cmd : Inport
  sensor : Inport  Port=2
  Constant : Constant  Value=Kp_T
  Constant1 : Constant  Value=Ki_T
  Constant2 : Constant  Value=Kd_T
  Data Type Conversion : DataTypeConversion
  PID : Subsystem
  Saturation : Saturate  UpperLimit=60  LowerLimit=-20
  Subsystem : Subsystem
  Sum : Sum  Inputs=|+-
  spring : Outport
  valve : Outport  Port=2
  wires:
  Constant1/1 -> PID/3(Ki)
  Constant2/1 -> PID/4(Kd)
  Constant/1 -> PID/2(Kp)
  Cmd/1 -> Saturation/1
  Subsystem/1(heating) -> spring/1
  Subsystem/2(cooling) -> valve/1
  Data Type Conversion/1 -> PID/1(e)
  Saturation/1 -> Sum/1
  sensor/1 -> Sum/2
  PID/1(u) -> Subsystem/1(u)
  Sum/1 -> Data Type Conversion/1

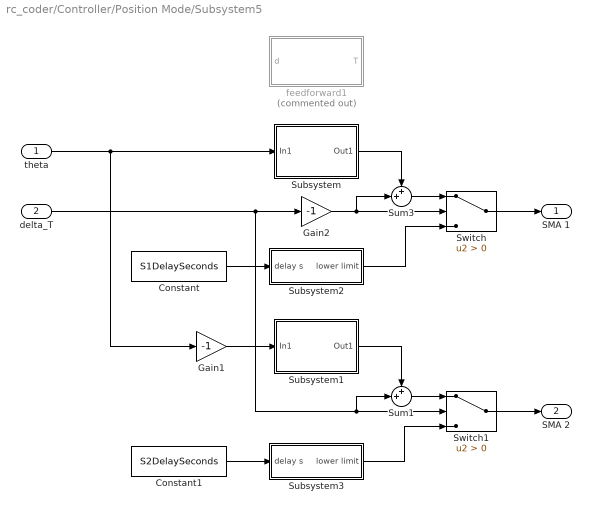
== system rc_coder/Controller/Position Mode/Subsystem5 ==
  theta : Inport
  delta_T : Inport  Port=2
  Constant : Constant  Value=S1DelaySeconds
  Constant1 : Constant  Value=S2DelaySeconds
  Gain1 : Gain  Gain=-1
  Gain2 : Gain  Gain=-1
  Subsystem : Subsystem
      mask Display: disp('feedforward\ncompensation');
  Subsystem1 : Subsystem
      mask Display: disp('feedforward\ncompensation');
  Subsystem2 : Subsystem
  Subsystem3 : Subsystem
  Sum1 : Sum  Inputs=++|
  Sum3 : Sum  Inputs=++|
  Switch : Switch  Criteria=u2 > Threshold
  Switch1 : Switch  Criteria=u2 > Threshold
  feedforward1 : Subsystem  Commented=on
      mask Display: disp('feedforward\ncompensation');
  SMA 1 : Outport
  SMA 2 : Outport  Port=2
  wires:
  delta_T/1 -> Gain2/1, Sum1/2, Switch1/2
  Switch/1 -> SMA 1/1
  Switch1/1 -> SMA 2/1
  Gain2/1 -> Sum3/2, Switch/2
  Sum3/1 -> Switch/1
  theta/1 -> Subsystem/1(In1), Gain1/1
  Subsystem/1(Out1) -> Sum3/1
  Sum1/1 -> Switch1/1
  Subsystem1/1(Out1) -> Sum1/1
  Gain1/1 -> Subsystem1/1(In1)
  Constant/1 -> Subsystem2/1(delay s)
  Constant1/1 -> Subsystem3/1(delay s)
  Subsystem3/1(lower limit) -> Switch1/3
  Subsystem2/1(lower limit) -> Switch/3

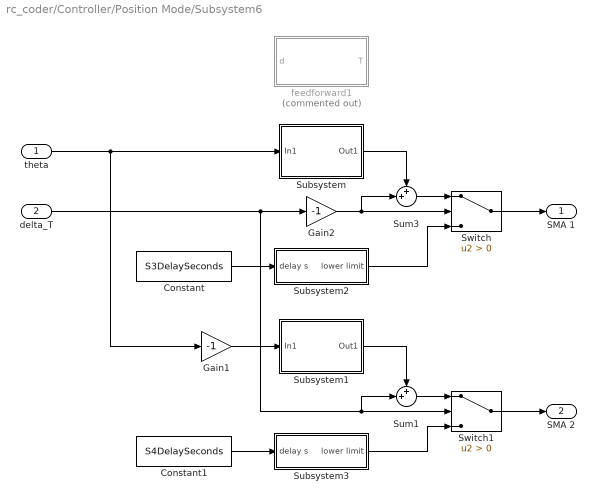
== system rc_coder/Controller/Position Mode/Subsystem6 ==
  theta : Inport
  delta_T : Inport  Port=2
  Constant : Constant  Value=S3DelaySeconds
  Constant1 : Constant  Value=S4DelaySeconds
  Gain1 : Gain  Gain=-1
  Gain2 : Gain  Gain=-1
  Subsystem : Subsystem
      mask Display: disp('feedforward\ncompensation');
  Subsystem1 : Subsystem
      mask Display: disp('feedforward\ncompensation');
  Subsystem2 : Subsystem
  Subsystem3 : Subsystem
  Sum1 : Sum  Inputs=++|
  Sum3 : Sum  Inputs=++|
  Switch : Switch  Criteria=u2 > Threshold
  Switch1 : Switch  Criteria=u2 > Threshold
  feedforward1 : Subsystem  Commented=on
      mask Display: disp('feedforward\ncompensation');
  SMA 1 : Outport
  SMA 2 : Outport  Port=2
  wires:
  Gain1/1 -> Subsystem1/1(In1)
  Subsystem1/1(Out1) -> Sum1/1
  Sum1/1 -> Switch1/1
  Subsystem/1(Out1) -> Sum3/1
  theta/1 -> Subsystem/1(In1), Gain1/1
  Sum3/1 -> Switch/1
  Gain2/1 -> Switch/2, Sum3/2
  Switch1/1 -> SMA 2/1
  Switch/1 -> SMA 1/1
  delta_T/1 -> Switch1/2, Sum1/2, Gain2/1
  Constant/1 -> Subsystem2/1(delay s)
  Subsystem3/1(lower limit) -> Switch1/3
  Constant1/1 -> Subsystem3/1(delay s)
  Subsystem2/1(lower limit) -> Switch/3

== system rc_coder/Controller/Temperature Mode/Subsystem1 ==
  Cmd : Inport
  sensor : Inport  Port=2
  Constant : Constant  Value=Kp_T
  Constant1 : Constant  Value=Ki_T
  Constant2 : Constant  Value=Kd_T
  Data Type Conversion : DataTypeConversion
  PID : Subsystem
  Saturation : Saturate  UpperLimit=60  LowerLimit=-20
  Subsystem : Subsystem
  Sum : Sum  Inputs=|+-
  spring : Outport
  valve : Outport  Port=2
  wires:
  Sum/1 -> Data Type Conversion/1
  PID/1(u) -> Subsystem/1(u)
  sensor/1 -> Sum/2
  Saturation/1 -> Sum/1
  Data Type Conversion/1 -> PID/1(e)
  Subsystem/2(cooling) -> valve/1
  Subsystem/1(heating) -> spring/1
  Cmd/1 -> Saturation/1
  Constant/1 -> PID/2(Kp)
  Constant2/1 -> PID/4(Kd)
  Constant1/1 -> PID/3(Ki)

== system rc_coder/Controller/Temperature Mode/Subsystem2 ==
  Cmd : Inport
  sensor : Inport  Port=2
  Constant : Constant  Value=Kp_T
  Constant1 : Constant  Value=Ki_T
  Constant2 : Constant  Value=Kd_T
  Data Type Conversion : DataTypeConversion
  PID : Subsystem
  Saturation : Saturate  UpperLimit=60  LowerLimit=-20
  Subsystem : Subsystem
  Sum : Sum  Inputs=|+-
  spring : Outport
  valve : Outport  Port=2
  wires:
  Constant1/1 -> PID/3(Ki)
  Constant2/1 -> PID/4(Kd)
  Constant/1 -> PID/2(Kp)
  Cmd/1 -> Saturation/1
  Subsystem/1(heating) -> spring/1
  Subsystem/2(cooling) -> valve/1
  Data Type Conversion/1 -> PID/1(e)
  Saturation/1 -> Sum/1
  sensor/1 -> Sum/2
  PID/1(u) -> Subsystem/1(u)
  Sum/1 -> Data Type Conversion/1

== system rc_coder/Controller/Temperature Mode/Subsystem3 ==
  Cmd : Inport
  sensor : Inport  Port=2
  Constant : Constant  Value=Kp_T
  Constant1 : Constant  Value=Ki_T
  Constant2 : Constant  Value=Kd_T
  Data Type Conversion : DataTypeConversion
  PID : Subsystem
  Saturation : Saturate  UpperLimit=60  LowerLimit=-20
  Subsystem : Subsystem
  Sum : Sum  Inputs=|+-
  spring : Outport
  valve : Outport  Port=2
  wires:
  Constant1/1 -> PID/3(Ki)
  Constant2/1 -> PID/4(Kd)
  Constant/1 -> PID/2(Kp)
  Cmd/1 -> Saturation/1
  Subsystem/1(heating) -> spring/1
  Subsystem/2(cooling) -> valve/1
  Data Type Conversion/1 -> PID/1(e)
  Saturation/1 -> Sum/1
  sensor/1 -> Sum/2
  PID/1(u) -> Subsystem/1(u)
  Sum/1 -> Data Type Conversion/1

== system rc_coder/Controller/Temperature Mode/Subsystem4 ==
  Cmd : Inport
  sensor : Inport  Port=2
  Constant : Constant  Value=Kp_T
  Constant1 : Constant  Value=Ki_T
  Constant2 : Constant  Value=Kd_T
  Data Type Conversion : DataTypeConversion
  PID : Subsystem
  Saturation : Saturate  UpperLimit=60  LowerLimit=-20
  Subsystem : Subsystem
  Sum : Sum  Inputs=|+-
  spring : Outport
  valve : Outport  Port=2
  wires:
  Sum/1 -> Data Type Conversion/1
  PID/1(u) -> Subsystem/1(u)
  sensor/1 -> Sum/2
  Saturation/1 -> Sum/1
  Data Type Conversion/1 -> PID/1(e)
  Subsystem/2(cooling) -> valve/1
  Subsystem/1(heating) -> spring/1
  Cmd/1 -> Saturation/1
  Constant/1 -> PID/2(Kp)
  Constant2/1 -> PID/4(Kd)
  Constant1/1 -> PID/3(Ki)

== system rc_coder/Controller/Temperature Mode/Subsystem5 ==
  Cmd : Inport
  sensor : Inport  Port=2
  Data Type Conversion : DataTypeConversion
  Discrete PID Controller : simulink/Continuous/PID Controller  Controller=PID  Form=Parallel  TimeDomain=Discrete-time  SampleTime=-1  IntegratorMethod=Forward Euler  FilterMethod=Forward Euler  ControllerParametersSource=internal  P=1.0  I=0.3  D=0.05  UseFilter=off  N=1  TunerSelectOption=Transfer Function Based (PID Tuner App)  InitialConditionSource=internal  InitialConditionForIntegrator=0  InitialConditionForFilter=0  DifferentiatorICPrevScaledInput=0  ExternalReset=none  TrackingMode=off  Kt=1  LimitOutput=off  UpperSaturationLimit=inf  LowerSaturationLimit=-inf  LinearizeAsGain=off  AntiWindupMode=none  Kb=1  POutMin=[]  POutMax=[]  IOutMin=[]  IOutMax=[]  DOutMin=[]  DOutMax=[]  NOutMin=[]  NOutMax=[]  SumOutMin=[]  SumOutMax=[]  SaturationOutMin=[]  SaturationOutMax=[]  PParamMin=[]  PParamMax=[]  IParamMin=[]  IParamMax=[]  DParamMin=[]  DParamMax=[]  NParamMin=[]  NParamMax=[]  KbParamMin=[]  KbParamMax=[]  KtParamMin=[]  KtParamMax=[]  KbOutMin=[]  KbOutMax=[]  KtOutMin=[]  KtOutMax=[]  IntegratorOutMin=[]  IntegratorOutMax=[]  FilterOutMin=[]  FilterOutMax=[]  SumI1OutMin=[]  SumI1OutMax=[]  SumI2OutMin=[]  SumI2OutMax=[]  SumI3OutMin=[]  SumI3OutMax=[]  SumI4OutMin=[]  SumI4OutMax=[]  SumDOutMin=[]  SumDOutMax=[]  DifferentiatorOutMin=[]  DifferentiatorOutMax=[]  FilterDiffOutCoefMin=[]  FilterDiffOutCoefMax=[]  ReciprocalOutMin=[]  ReciprocalOutMax=[]  SumDenOutMin=[]  SumDenOutMax=[]  SumNumOutMin=[]  SumNumOutMax=[]  DivideOutMin=[]  DivideOutMax=[]  IntegratorContinuousStateAttributes=''  IntegratorStateMustResolveToSignalObject=off  IntegratorRTWStateStorageClass=Auto  FilterContinuousStateAttributes=''  FilterStateMustResolveToSignalObject=off  FilterRTWStateStorageClass=Auto  ParallelPVariant=InternalParameters  IdealPVariant=Disabled  IVariant=InternalParameters  DVariant=InternalParameters  IntegratorVariant=Discrete  SatVariant=Disabled  AWVariant=Passthrough  PCopyVariant=Disabled  TRVariant=Disabled  FdbkBlocksVariant=Forward  IdealPFdbkVariant=Disabled  SatFdbkVariant=Disabled  DerivativeFilterVariant=Differentiator  NVariant=Passthrough  NCopyVariant=Disabled_SignalSpec  FilterICVariant=InternalICsDifferentiator  IntegratorICVariant=InternalICs  ExternalResetVariant=Disabled  TRSumVariant=Passthrough  SumFdbkVariant=Disabled  SumVariant=Sum_PID
  PID_1 : Subsystem
  Saturation : Saturate  UpperLimit=60  LowerLimit=-20
  Subsystem : Subsystem
  Sum : Sum  Inputs=|+-
  spring : Outport
  valve : Outport  Port=2
  wires:
  Cmd/1 -> Saturation/1
  Subsystem/1(heating) -> spring/1
  Subsystem/2(cooling) -> valve/1
  Data Type Conversion/1 -> Discrete PID Controller/1
  Saturation/1 -> Sum/1
  sensor/1 -> Sum/2
  Discrete PID Controller/1 -> Subsystem/1(u)
  Sum/1 -> Data Type Conversion/1

== system rc_coder/DataComposer/ElapsedTime/Triggered Subsystem ==
  In1 : Inport
  Trigger : TriggerPort  TriggerType=falling  VariantControl=Variant
  Increment Real World : simulink/Additional Math & Discrete/Additional Math: Increment - Decrement/Increment Real World
      settings: SourceProductName=Simulink  SourceProductBaseCode=SL
  Out1 : Outport
  wires:
  In1/1 -> Increment Real World/1
  Increment Real World/1 -> Out1/1

== system rc_coder/Sensing/Current Measurement/adc2current ==
  adc_voltage : Inport
  Constant : Constant  Value=ADCDRES / 2
  Gain4 : Gain  Gain=VADCREF / ADCDRES / SamplingR
  Subtract : Sum  Inputs=+-
  current : Outport
  wires:
  adc_voltage/1 -> Subtract/1
  Constant/1 -> Subtract/2
  Gain4/1 -> current/1
  Subtract/1 -> Gain4/1

== system rc_coder/Sensing/Current Measurement/adc2current1 ==
  adc_voltage : Inport
  Constant : Constant  Value=ADCDRES / 2
  Gain4 : Gain  Gain=VADCREF / ADCDRES / SamplingR
  Subtract : Sum  Inputs=+-
  current : Outport
  wires:
  Subtract/1 -> Gain4/1
  Gain4/1 -> current/1
  Constant/1 -> Subtract/2
  adc_voltage/1 -> Subtract/1

== system rc_coder/Sensing/Current Measurement/adc2current2 ==
  adc_voltage : Inport
  Constant : Constant  Value=ADCDRES / 2
  Gain4 : Gain  Gain=VADCREF / ADCDRES / SamplingR
  Subtract : Sum  Inputs=+-
  current : Outport
  wires:
  adc_voltage/1 -> Subtract/1
  Constant/1 -> Subtract/2
  Gain4/1 -> current/1
  Subtract/1 -> Gain4/1

== system rc_coder/Sensing/Current Measurement/adc2current3 ==
  adc_voltage : Inport
  Constant : Constant  Value=ADCDRES / 2
  Gain4 : Gain  Gain=VADCREF / ADCDRES / SamplingR
  Subtract : Sum  Inputs=+-
  current : Outport
  wires:
  Subtract/1 -> Gain4/1
  Gain4/1 -> current/1
  Constant/1 -> Subtract/2
  adc_voltage/1 -> Subtract/1

== system rc_coder/Sensing/Incremental Encoder/CalcSpd ==
  dir : Inport
  qposcnt : Inport  Port=2
  qcprd : Inport  Port=3
  overflow : Inport  Port=4
  Constant6 : Constant  Value=0
  Divide1 : Product  Inputs=**
  Lowpass Filter : dspfdesign/Lowpass Filter  FilterType=FIR  DesignForMinimumOrder=on  FilterOrder=50  PassbandFrequency=20  StopbandFrequency=200  PassbandRipple=0.1  StopbandAttenuation=80  InheritSampleRate=off  SampleRate=1e3  SimulateUsing=Code generation  roundingMode=Floor  coeffsDataTypeStr=fixdt(1,16)
  OF_Initial_check : Subsystem
  Switch4 : Switch  Criteria=u2 ~= 0
  cnt2rpm : Subsystem
  dir_check : Subsystem
  zero_spd_check : Subsystem
  speed : Outport
  wires:
  qcprd/1 -> OF_Initial_check/2(cnt_prd), cnt2rpm/1(cnt_prd)
  Divide1/1 -> Switch4/3
  Switch4/1 -> Lowpass Filter/1
  Constant6/1 -> Switch4/1
  qposcnt/1 -> zero_spd_check/1(poscnt)
  zero_spd_check/1(flag) -> Switch4/2
  dir/1 -> dir_check/1(dir_flag)
  dir_check/1(dir) -> Divide1/1
  cnt2rpm/1(radps) -> OF_Initial_check/1(spd_in)
  overflow/1 -> OF_Initial_check/3(OF_flag)
  OF_Initial_check/1(spd_out) -> zero_spd_check/2(last_measurement), Divide1/2
  Lowpass Filter/1 -> speed/1

== system rc_coder/Sensing/Incremental Encoder/CalcSpd1 ==
  dir : Inport
  qposcnt : Inport  Port=2
  qcprd : Inport  Port=3
  overflow : Inport  Port=4
  Constant6 : Constant  Value=0
  Divide1 : Product  Inputs=**
  Lowpass Filter : dspfdesign/Lowpass Filter  FilterType=FIR  DesignForMinimumOrder=on  FilterOrder=50  PassbandFrequency=20  StopbandFrequency=200  PassbandRipple=0.1  StopbandAttenuation=80  InheritSampleRate=off  SampleRate=1e3  SimulateUsing=Code generation  roundingMode=Floor  coeffsDataTypeStr=fixdt(1,16)
  OF_Initial_check : Subsystem
  Switch4 : Switch  Criteria=u2 ~= 0
  cnt2rpm : Subsystem
  dir_check : Subsystem
  zero_spd_check : Subsystem
  speed : Outport
  wires:
  Lowpass Filter/1 -> speed/1
  OF_Initial_check/1(spd_out) -> Divide1/2, zero_spd_check/2(last_measurement)
  overflow/1 -> OF_Initial_check/3(OF_flag)
  cnt2rpm/1(radps) -> OF_Initial_check/1(spd_in)
  dir_check/1(dir) -> Divide1/1
  dir/1 -> dir_check/1(dir_flag)
  zero_spd_check/1(flag) -> Switch4/2
  qposcnt/1 -> zero_spd_check/1(poscnt)
  Constant6/1 -> Switch4/1
  Switch4/1 -> Lowpass Filter/1
  Divide1/1 -> Switch4/3
  qcprd/1 -> cnt2rpm/1(cnt_prd), OF_Initial_check/2(cnt_prd)
